simulink model "AD1939_Avalon_Stream_Processing_v1"  (R2018b)
settings: Solver=FixedStepDiscrete  StartTime=0.0  StopTime=stop_time  RelTol=1e-3
InitFcn:
  | DataPlane_callback_init
StopFcn:
  | DataPlane_callback_stop
undefined symbols (not defined in the file or in its folder): F_bits, Ts_system, W_bits
libraries: hdlsllib x18, simulink x5, dspsrcs4 x4, dsphdlfiltering x2
(part 2 of 2)

== stateflow chart AD1939_Avalon_Stream_Processing_v1/DataPlane/Signal Energy LED Driver/Left Channel Processing/LED_Driver/Subsystem6/Chart ==
  settings: executeAtInitialization=1
  note: Turn on LED (LED_signal = true)
      | and start the counter when the LED_on state is entered.
      | When the counter reaches final count value, count_reach is asserted and
      | the state transitions to LED_off where the LED is turned off.
  state LED_on
    entry: LED_signal=true;
    entry: counter_reset=false;
  state LED_off
    entry: LED_signal=false;
    entry: counter_reset=true;
  note: Transition to state LED_on
      | when LED_trigger is asserted
  note: To update, parse chart to update signal names
      | Chart -> Parse Chart
      |
      | To add/remove/edit signals see:
      |  https://www.mathworks.com/help/stateflow/ug/using-the-model-explorer-with-stateflow-objects.html
  (default) -> LED_off
  LED_off -> LED_on : [LED_trigger == 1]
  LED_on -> LED_off [order 2] : [count_reached==1]
  LED_on -> LED_on [order 1] : [count_reached == 0]
  data: LED_trigger input; count_reached input; LED_signal output; counter_reset output

== stateflow chart AD1939_Avalon_Stream_Processing_v1/DataPlane/Signal Energy LED Driver/Left Channel Processing/LED_Driver/Subsystem7/Chart ==
  settings: executeAtInitialization=1
  note: Turn on LED (LED_signal = true)
      | and start the counter when the LED_on state is entered.
      | When the counter reaches final count value, count_reach is asserted and
      | the state transitions to LED_off where the LED is turned off.
  state LED_on
    entry: LED_signal=true;
    entry: counter_reset=false;
  state LED_off
    entry: LED_signal=false;
    entry: counter_reset=true;
  note: Transition to state LED_on
      | when LED_trigger is asserted
  note: To update, parse chart to update signal names
      | Chart -> Parse Chart
      |
      | To add/remove/edit signals see:
      |  https://www.mathworks.com/help/stateflow/ug/using-the-model-explorer-with-stateflow-objects.html
  (default) -> LED_off
  LED_off -> LED_on : [LED_trigger == 1]
  LED_on -> LED_off [order 2] : [count_reached==1]
  LED_on -> LED_on [order 1] : [count_reached == 0]
  data: LED_trigger input; count_reached input; LED_signal output; counter_reset output
